simulink model "platooning_sim"  (R2022a)
settings: Solver=VariableStepAuto  StartTime=0.0  StopTime=10  RelTol=1e-3
libraries: simulink x2
settings Model: Creator=david  LastModifiedBy=david

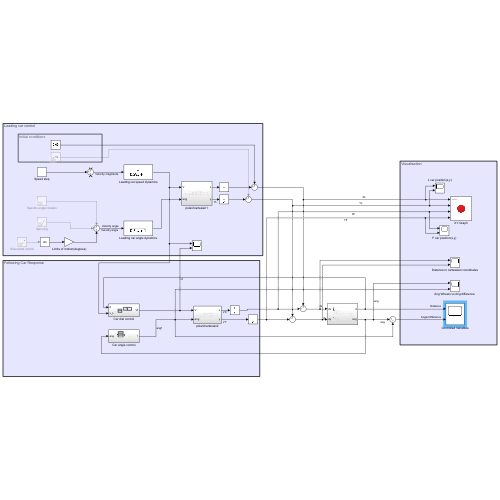
[thumbnail: Simulink's stored preview of the top-level diagram]
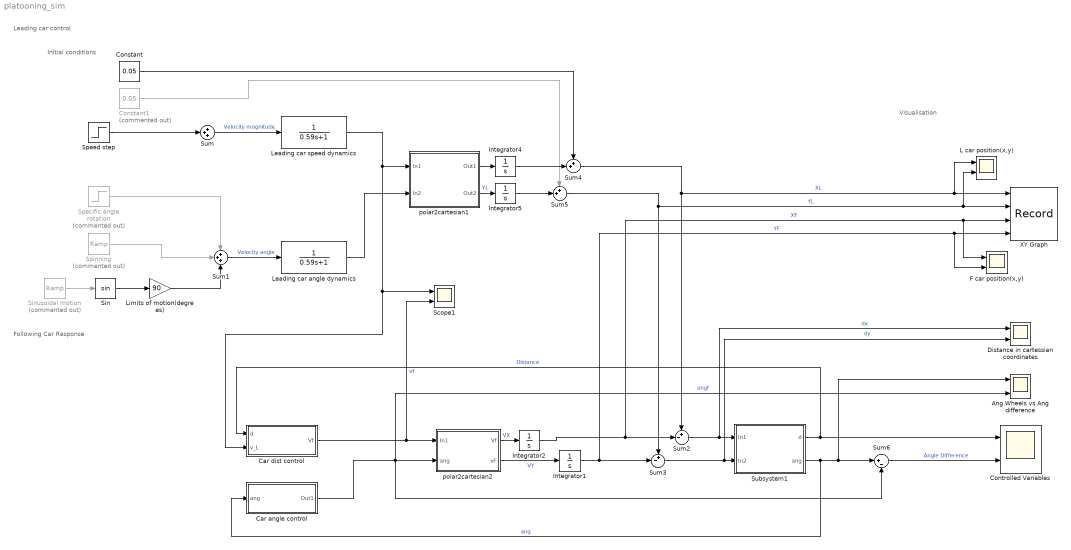
== system platooning_sim ==
  note: Visualisation
  note: Initial conditions
  note: Following Car Response
  note: Leading car control
  "Ang Wheels vs Ang difference " : Scope  NumInputPorts=2
  Car angle control : Subsystem
  Car dist control : Subsystem
  Constant : Constant  Value=0.05
  Constant1 : Constant  Commented=on  Value=0.05
  Controlled Variables : Scope  NumInputPorts=2
  Distance in cartessian coordinates : Scope  NumInputPorts=2
  F car position(x,y) : Scope  NumInputPorts=2
  Integrator{1..2,4..5} (4 alike) : Integrator
  L car position(x,y) : Scope  NumInputPorts=2
  Leading car angle dynamics : TransferFcn  Denominator=[0.59 1]
  Leading car speed dynamics : TransferFcn  Denominator=[0.59 1]
  Limits of motion(degrees) : Gain  Gain=90
  Scope1 : Scope  NumInputPorts=2
  Sin : Trigonometry
  Sinusoidal motion : simulink/Sources/Ramp  Commented=on  slope=pi  start=0  InitialOutput=0
  Specific angle rotation : Step  Commented=on  Time=3  After=5  SampleTime=0
  Speed step : Step  Time=0  After=10  SampleTime=1
  Spinning : simulink/Sources/Ramp  Commented=on  slope=5*180/pi  start=0  InitialOutput=0
  Subsystem1 : Subsystem
  Sum : Sum  Inputs=+++
  Sum1 : Sum  Inputs=+++
  Sum2 : Sum  Inputs=+-|
  Sum3 : Sum  Inputs=+-|
  Sum4 : Sum  Inputs=++|
  Sum5 : Sum  Inputs=++|
  Sum6 : Sum  Inputs=|+-
  XY Graph : Record  FileSettingsInternal="{\"entries\":[{\"content\":{\"excelSettings\":{\"content\":{},\"type\":\"Streamout.ExcelSettings\"}},\"type\":\"Streamout.FileSettingStorage\",\"uuid\":\"1f241d09-22e1-462e-9762-0058fec7610a\"}],\"packageUris\":[\"http://schema.mathworks.com/mf0/streamout_blocks/R2020a\"],\"version\":\"1.0\"}"  Layout=[1 1]  SignalsInternal="{\"entries\":[{\"content\":{\"signals\":[{\"content\":{\"blockPath\":[\"platooning_sim/XY Graph\"],\"channel\":[],\"dimensions\":[1],\"domain\":\"platooning_sim/XY Graph\",\"lineColor\":\"#a2142f\",\"plots\":[1],\"port\":1,\"sid\":[\"\"],\"signalID\":235,\"signalName\":\"XL\"},\"type\":\"RecordBlkView.Signal\",\"uuid\":\"b307e947-2b89-47f2-ab75-c2c398885e15\"},{\"content\":{\"blockPath\":[\"platooning_sim/XY Graph\"],\"channel\":[],\"dimensions\":[1],\"domain\":\"platooning_sim/XY Graph\",\"lineColor\":\"#139fff\",\"plots\":[1],\"port\":2,\"sid\":[\"\"],\"signalID\":239,\"signalName\":\"YL\"},\"type\":\"RecordBlkView.Signal\",\"uuid\":\"444089d4-2c3a-42a8-a449-182ef98061f8\"},{\"content\":{\"blockPath\":[\"platooning_sim/XY Graph\"],\"channel\":[],\"dimensions\":[1],\"domain\":\"platooning_sim/XY Graph\",\"lineColor\":\"#64d413\",\"plots\":[1],\"port\":3,\"sid\":[\"\"],\"signalID\":243,\"signalName\":\"XF\"},\"type\":\"RecordBlkView.Signal\",\"uuid\":\"c3651b09-46f7-4a26-9e1b-4184f1efad10\"},{\"content\":{\"blockPath\":[\"platooning_sim/XY Graph\"],\"channel\":[],\"dimensions\":[1],\"domain\":\"platooning_sim/XY Graph\",\"lineColor\":\"#ff13a6\",\"plots\":[1],\"port\":4,\"sid\":[\"\"],\"signalID\":247,\"signalName\":\"YF\"},\"type\":\"RecordBlkView.Signal\",\"uuid\":\"099ca2ec-3b9f-40ce-9790-c88963085856\"}]},\"type\":\"RecordBlkView.InputSignals\",\"uuid\":\"64080609-3876-47d6-8f69-335b8658d89f\"}],\"packageUris\":[\"http://schema.mathworks.com/mf0/streamout_blocks/R2020a\"],\"version\":\"1.0\"}"  VisualizationBindings="{\"xyplotplugin\":{\"info\":[{\"series\":[{\"bindingParametersList\":[{\"parameter\":\"X-Axis\",\"signalID\":235,\"signalName\":\"XL\"},{\"parameter\":\"Y-Axis\",\"signalID\":239,\"signalName\":\"YL\"}],\"seriesID\":56638},{\"bindingParametersList\":[{\"parameter\":\"X-Axis\",\"signalID\":243,\"signalName\":\"XF\"},{\"parameter\":\"Y-Axis\",\"signalID\":247,\"signalName\":\"YF\"}],\"seriesID\":17436}],\"subplotID\":1}]}}"  CompatibilityTag=XY
  polar2cartesian1 : Subsystem
  polar2cartesian2 : Subsystem
  wires:
  Speed step/1 -> Sum/2
  Sum/1 -> Leading car speed dynamics/1  "Velocity magnitude"
  Sum1/1 -> Leading car angle dynamics/1  "Velocity angle"
  polar2cartesian2/1(Vf) -> Integrator2/1  "VX"
  Sum5/1 -> Sum3/1, L car position(x,y)/2, XY Graph/2  "YL"
  polar2cartesian2/2(vF) -> Integrator1/1  "VY"
  Subsystem1/1(d) -> Car dist control/1(d), Controlled Variables/1  "Distance"
  polar2cartesian1/1(Out1) -> Integrator4/1
  Sum4/1 -> Sum2/1, L car position(x,y)/1, XY Graph/1  "XL"
  Constant/1 -> Sum4/1
  Sum2/1 -> Distance in cartessian coordinates/1, Subsystem1/1(In1)  "dx"
  Sum3/1 -> Distance in cartessian coordinates/2, Subsystem1/2(In2)  "dy"
  Subsystem1/2(ang) -> "Ang Wheels vs Ang difference "/1, Sum6/1, Car angle control/1(ang)  "ang"
  Specific angle rotation/1 -> Sum1/1
  Car dist control/1(Vf) -> Scope1/2, polar2cartesian2/1(In1)  "vf"
  polar2cartesian1/2(Out2) -> Integrator5/1  "YL"
  Constant1/1 -> Sum5/1
  Car angle control/1(Out1) -> polar2cartesian2/2(ang), Sum6/2, "Ang Wheels vs Ang difference "/2  "angf"
  Integrator1/1 -> F car position(x,y)/2, XY Graph/4, Sum3/2  "YF"
  Integrator2/1 -> F car position(x,y)/1, XY Graph/3, Sum2/2  "XF"
  Integrator4/1 -> Sum4/2
  Integrator5/1 -> Sum5/2
  Leading car speed dynamics/1 -> Scope1/1, Car dist control/2(v_L), polar2cartesian1/1(In1)
  Leading car angle dynamics/1 -> polar2cartesian1/2(In2)
  Sum6/1 -> Controlled Variables/2  "Angle Difference"
  Sinusoidal motion/1 -> Sin/1
  Sin/1 -> Limits of motion(degrees)/1
  Limits of motion(degrees)/1 -> Sum1/3
  Spinning/1 -> Sum1/2

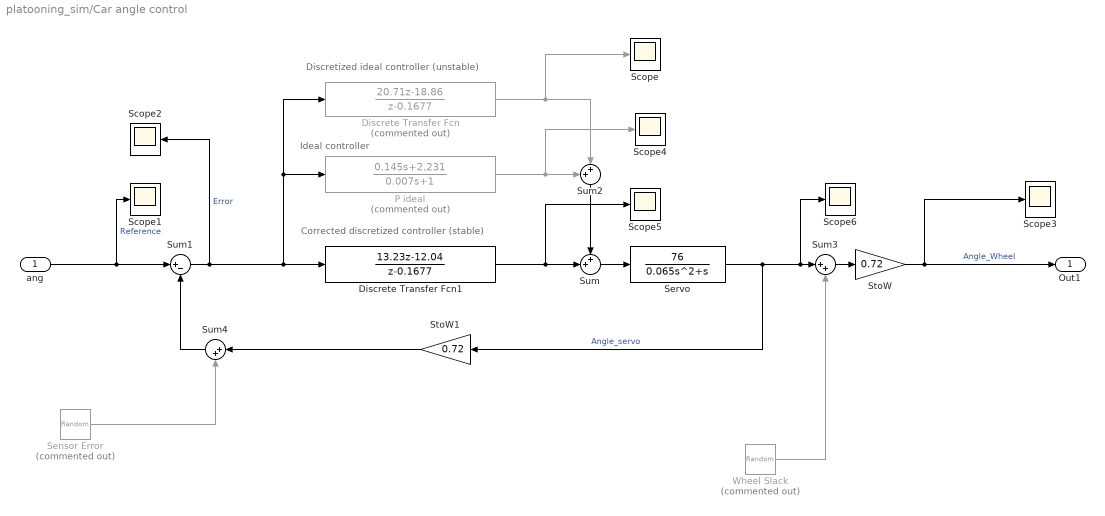
== system platooning_sim/Car angle control ==
  note: Discretized ideal controller (unstable)
  note: Ideal controller
  note: Corrected discretized controller (stable)
  ang : Inport
  Discrete Transfer Fcn : DiscreteTransferFcn  Commented=on  Numerator=[20.71 -18.86]  Denominator=[1 -0.1677]  SampleTime=1/80
  Discrete Transfer Fcn1 : DiscreteTransferFcn  Numerator=[13.23 -12.04]  Denominator=[1 -0.1677]  SampleTime=1/80
  P ideal : TransferFcn  Commented=on  Numerator=[0.145 2.231]  Denominator=[0.007 1]
  Scope{,1..6} (7 alike) : Scope
  Sensor Error : RandomNumber  Commented=on  Variance=4  SampleTime=1/80
  Servo : TransferFcn  Numerator=[76]  Denominator=[0.065 1 0]
  StoW : Gain  Gain=0.72
  StoW1 : Gain  Gain=0.72
  Sum : Sum  Inputs=++|
  Sum1 : Sum  Inputs=|+-
  Sum2 : Sum  Inputs=++|
  Sum3 : Sum  Inputs=|++
  Sum4 : Sum  Inputs=|++
  Wheel Slack : RandomNumber  Commented=on  Variance=3  Seed=123123  SampleTime=0.001
  Out1 : Outport
  wires:
  StoW/1 -> Scope3/1, Out1/1  "Angle_Wheel"
  Servo/1 -> StoW1/1, Sum3/1, Scope6/1  "Angle_servo"
  StoW1/1 -> Sum4/1
  ang/1 -> Sum1/1, Scope1/1  "Reference"
  Sum1/1 -> Discrete Transfer Fcn/1, P ideal/1, Discrete Transfer Fcn1/1, Scope2/1  "Error"
  Discrete Transfer Fcn1/1 -> Scope5/1, Sum/2
  Sum2/1 -> Sum/1
  Sum/1 -> Servo/1
  P ideal/1 -> Scope4/1, Sum2/1
  Discrete Transfer Fcn/1 -> Scope/1, Sum2/2
  Sum3/1 -> StoW/1
  Sum4/1 -> Sum1/2
  Sensor Error/1 -> Sum4/2
  Wheel Slack/1 -> Sum3/2

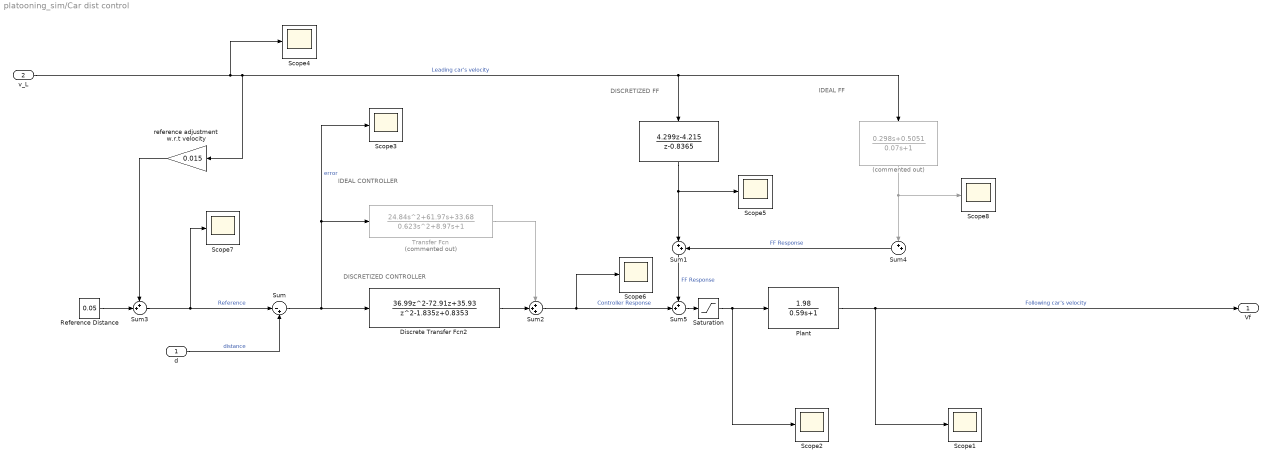
== system platooning_sim/Car dist control ==
  note: IDEAL CONTROLLER
  note: DISCRETIZED CONTROLLER
  note: IDEAL FF
  note: DISCRETIZED FF
  d : Inport
  v_L : Inport  Port=2
  " " : TransferFcn  Commented=on  Numerator=[0.298 0.5051]  Denominator=[0.07 1]
  "  " : DiscreteTransferFcn  Numerator=[4.299 -4.215]  Denominator=[1 -0.8365]  SampleTime=1/80
  Discrete Transfer Fcn2 : DiscreteTransferFcn  Numerator=[36.99 -72.91 35.93]  Denominator=[1 -1.835 0.8353]  SampleTime=1/80
  Plant : TransferFcn  Numerator=[1.98]  Denominator=[0.59 1]
  Reference Distance : Constant  Value=0.05
  Saturation : Saturate  UpperLimit=8  LowerLimit=-8
  Scope{1..8} (8 alike) : Scope
  Sum : Sum  Inputs=|-+
  Sum1 : Sum  Inputs=|++
  Sum2 : Sum  Inputs=+++
  Sum3 : Sum  Inputs=++|
  Sum4 : Sum  Inputs=++|
  Sum5 : Sum  Inputs=++|
  Transfer Fcn : TransferFcn  Commented=on  Numerator=[24.84 61.97 33.68]  Denominator=[0.623 8.97 1]
  reference adjustment w.r.t velocity : Gain  Gain=0.015
  Vf : Outport
  wires:
  Reference Distance/1 -> Sum3/2
  Sum5/1 -> Saturation/1
  reference adjustment w.r.t velocity/1 -> Sum3/1
  Saturation/1 -> Scope2/1, Plant/1
  "  "/1 -> Sum1/1, Scope5/1
  Sum3/1 -> Sum/1, Scope7/1  "Reference"
  Plant/1 -> Vf/1, Scope1/1  "Following car's velocity"
  d/1 -> Sum/2  "distance"
  Sum/1 -> Scope3/1, Transfer Fcn/1, Discrete Transfer Fcn2/1  "error"
  Sum1/1 -> Sum5/1  "FF Response"
  " "/1 -> Scope8/1, Sum4/1
  Discrete Transfer Fcn2/1 -> Sum2/2
  Sum2/1 -> Scope6/1, Sum5/2  "Controller Response"
  Transfer Fcn/1 -> Sum2/1
  v_L/1 -> " "/1, "  "/1, reference adjustment w.r.t velocity/1, Scope4/1  "Leading car's velocity"
  Sum4/1 -> Sum1/2  "FF Response"

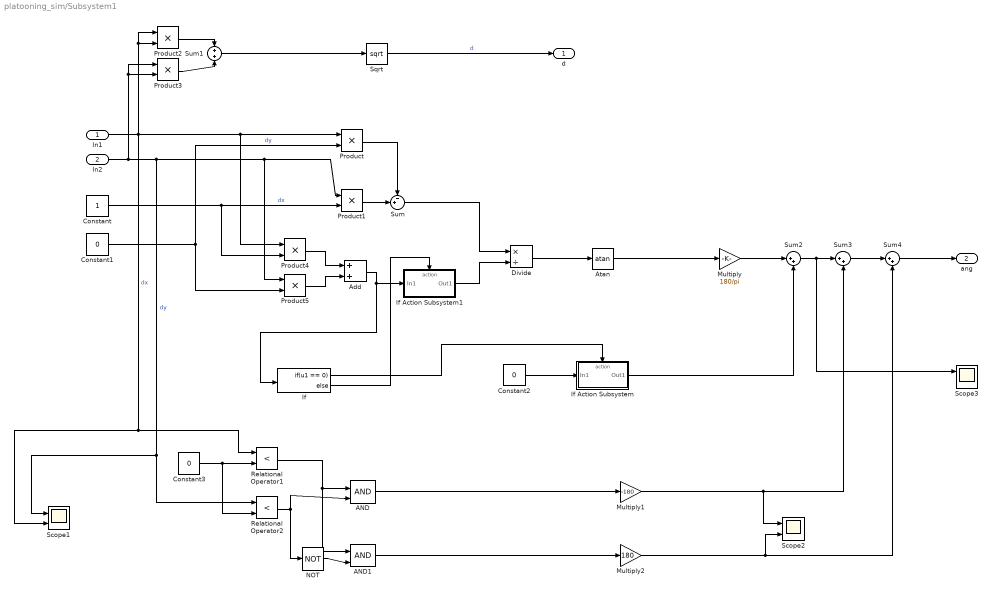
== system platooning_sim/Subsystem1 ==
  In1 : Inport
  In2 : Inport  Port=2
  AND : Logic  IconShape=distinctive  AllPortsSameDT=off  OutDataTypeStr=boolean
  AND1 : Logic  IconShape=distinctive  AllPortsSameDT=off  OutDataTypeStr=boolean
  Add : Sum
  Atan : Trigonometry  Operator=atan
  Constant : Constant
  Constant1 : Constant  Value=0
  Constant2 : Constant  Value=0
  Constant3 : Constant  Value=0
  Divide : Product  Inputs=*/
  If : If  IfExpression=u1 == 0
  If Action Subsystem : Subsystem  TreatAsAtomicUnit=on
  If Action Subsystem1 : Subsystem  TreatAsAtomicUnit=on
  Multiply : Gain  Gain=180/pi
  Multiply1 : Gain  Gain=-180
  Multiply2 : Gain  Gain=180
  NOT : Logic  Operator=NOT  IconShape=distinctive  AllPortsSameDT=off  OutDataTypeStr=boolean
  Product{,1..5} (6 alike) : Product
  Relational Operator1 : RelationalOperator  Operator=<  RndMeth=Simplest  InputSameDT=off
  Relational Operator2 : RelationalOperator  Operator=<  RndMeth=Simplest  InputSameDT=off
  Scope1 : Scope  NumInputPorts=2
  Scope2 : Scope  NumInputPorts=2
  Scope3 : Scope  NumInputPorts=2
  Sqrt : Sqrt
  Sum : Sum  Inputs=-+|
  Sum1 : Sum  Inputs=+|+
  Sum2 : Sum  Inputs=|++
  Sum3 : Sum  Inputs=|++
  Sum4 : Sum  Inputs=|++
  d : Outport
  ang : Outport  Port=2
  wires:
  In1/1 -> Relational Operator1/1, Scope1/2, Product2/2, Product2/1, Product4/1, Product/1  "dx"
  Constant/1 -> Product4/2, Product1/2  "dx"
  Constant1/1 -> Product/2, Product5/2  "dy"
  Sum1/1 -> Sqrt/1
  Sum/1 -> Divide/1
  Divide/1 -> Atan/1
  Atan/1 -> Multiply/1
  Sqrt/1 -> d/1  "d"
  Product1/1 -> Sum/2
  Product/1 -> Sum/1
  In2/1 -> Relational Operator2/1, Scope1/1, Product5/1, Product1/1, Product3/2, Product3/1  "dy"
  Product2/1 -> Sum1/1
  Product3/1 -> Sum1/2
  Product4/1 -> Add/1
  Product5/1 -> Add/2
  Add/1 -> If Action Subsystem1/1(In1), If/1
  If/1 -> If Action Subsystem/Action
  Constant2/1 -> If Action Subsystem/1(In1)
  Multiply/1 -> Sum2/1
  If Action Subsystem/1(Out1) -> Sum2/2
  If Action Subsystem1/1(Out1) -> Divide/2
  If/2 -> If Action Subsystem1/Action
  Sum2/1 -> Scope3/1, Sum3/1
  Sum3/1 -> Sum4/1
  Sum4/1 -> ang/1
  Constant3/1 -> Relational Operator2/2, Relational Operator1/2
  Relational Operator1/1 -> AND1/1, AND/1
  Relational Operator2/1 -> NOT/1, AND/2
  NOT/1 -> AND1/2
  AND/1 -> Multiply1/1
  AND1/1 -> Multiply2/1
  Multiply1/1 -> Scope2/1, Sum3/2
  Multiply2/1 -> Scope2/2, Sum4/2

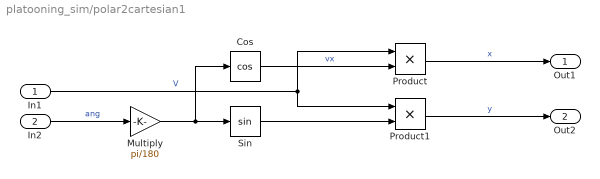
== system platooning_sim/polar2cartesian1 ==
  In1 : Inport
  In2 : Inport  Port=2
  Cos : Trigonometry  Operator=cos
  Multiply : Gain  Gain=pi/180
  Product : Product
  Product1 : Product
  Sin : Trigonometry
  Out1 : Outport
  Out2 : Outport  Port=2
  wires:
  In1/1 -> Product/1, Product1/1  "V"
  In2/1 -> Multiply/1  "ang"
  Cos/1 -> Product/2  "vx"
  Product1/1 -> Out2/1  "y"
  Sin/1 -> Product1/2
  Multiply/1 -> Sin/1, Cos/1
  Product/1 -> Out1/1  "x"

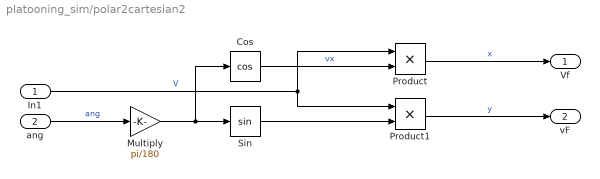
== system platooning_sim/polar2cartesian2 ==
  In1 : Inport
  ang : Inport  Port=2
  Cos : Trigonometry  Operator=cos
  Multiply : Gain  Gain=pi/180
  Product : Product
  Product1 : Product
  Sin : Trigonometry
  Vf : Outport
  vF : Outport  Port=2
  wires:
  In1/1 -> Product/1, Product1/1  "V"
  ang/1 -> Multiply/1  "ang"
  Cos/1 -> Product/2  "vx"
  Product1/1 -> vF/1  "y"
  Sin/1 -> Product1/2
  Multiply/1 -> Sin/1, Cos/1
  Product/1 -> Vf/1  "x"

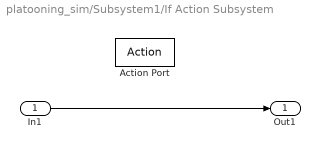
== system platooning_sim/Subsystem1/If Action Subsystem ==
  In1 : Inport
  Action Port : ActionPort  ActionPortLabel=if(u1 == 0)
  Out1 : Outport
  wires:
  In1/1 -> Out1/1

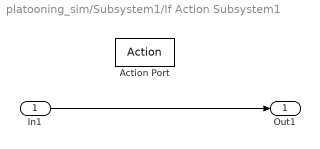
== system platooning_sim/Subsystem1/If Action Subsystem1 ==
  In1 : Inport
  Action Port : ActionPort  ActionPortLabel=else
  Out1 : Outport
  wires:
  In1/1 -> Out1/1
